simulink model "SMC_for_takeoff"  (R2018b)
settings: Solver=ode45  StartTime=0.0  StopTime=10.0  RelTol=1e-3
libraries: simulink x3
settings Model: Creator=mchehadeh  LastModifiedBy=aaa_b
settings DataIOCC: LimitDataPoints=on  SaveFormat=Array  SignalLoggingSaveFormat=ModelDataLogs
settings OptimizationCC: BlockReduction=off  BooleanDataType=off  ExpressionDepthLimit=2147483647  LifeSpan=inf
settings DebuggingCC: SaveWithParameterizedLinksMsg=none  UnderspecifiedInitializationDetection=Classic  MergeDetectMultiDrivingBlocksExec=none  SignalResolutionControl=TryResolveAllWithWarning  MultiTaskDSMMsg=warning  MultiTaskCondExecSysMsg=none  StateNameClashWarn=warning  SFUnexpectedBacktrackingDiag=warning  SFNoUnconditionalDefaultTransitionDiag=warning  SFExecutionAtInitializationDiag=none
settings HardwareCC: ProdBitPerPointer=32  ProdBitPerSizeT=32  ProdBitPerPtrDiffT=32  ProdLargestAtomicFloat=None  ProdIntDivRoundTo=Undefined  ProdEndianess=Unspecified  ProdWordSize=32  ProdHWDeviceType=32-bit Generic  TargetUnknown=on
settings ModelReferenceCC: PropagateSignalLabelsOutOfModel=off
settings SFSimCC: SimUseLocalCustomCode=off
settings RTWCC: RTWUseLocalCustomCode=off
settings CodeAppCC: StateflowObjectComments=on
settings GRTTargetCC: TargetLangStandard=C89/C90 (ANSI)  GeneratePreprocessorConditionals=Disable all
settings ConfigComp: CovMetricSettings=dw  CovHtmlReporting=on  CovSaveCumulativeToWorkspaceVar=on  CovSaveSingleToWorkspaceVar=on  CovExternalEMLEnable=off

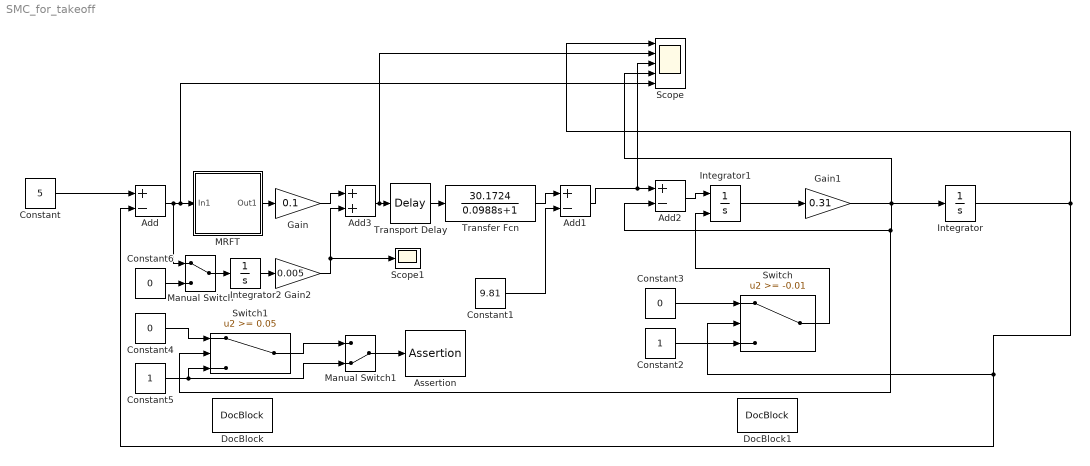
== system SMC_for_takeoff ==
  Add : Sum  Inputs=+-
  Add1 : Sum  Inputs=+-
  Add2 : Sum  Inputs=+-
  Add3 : Sum
  Assertion : Assertion  AssertionFailFcn=|  StopWhenAssertionFail=off
      | set_param(bdroot,'SimulationCommand','pause'),
      | disp(sprintf('\nSimulation paused.'))
  Constant : Constant  Value=5
  Constant1 : Constant  Value=9.81
  Constant2 : Constant
  Constant3 : Constant  Value=0
  Constant4 : Constant  Value=0
  Constant5 : Constant
  Constant6 : Constant  Value=0
  DocBlock : simulink/Model-Wide Utilities/DocBlock  DocumentType=Text
  DocBlock1 : simulink/Model-Wide Utilities/DocBlock  DocumentType=Text
  Gain : Gain  Gain=0.1
  Gain1 : Gain  Gain=0.31
  Gain2 : Gain  Gain=0.005
  Integrator : Integrator  LimitOutput=on  LowerSaturationLimit=0
  Integrator1 : Integrator  ExternalReset=level  LowerSaturationLimit=0
  Integrator2 : Integrator
  MRFT : Subsystem
  Manual Switch : ManualSwitch
  Manual Switch1 : ManualSwitch  CurrentSetting=0
  Scope : Scope  NumInputPorts=5
  Scope1 : Scope
  Switch : Switch  Threshold=-0.01
  Switch1 : Switch  Threshold=0.05
  Transfer Fcn : TransferFcn  Numerator=[30.1724]  Denominator=[0.0988 1]
  Transport Delay : TransportDelay  DelayTime=0.0709
  wires:
  Transport Delay/1 -> Transfer Fcn/1
  Integrator/1 -> Switch/2, Add/2, Scope/1
  MRFT/1(Out1) -> Gain/1
  Transfer Fcn/1 -> Add1/1
  Constant/1 -> Add/1
  Constant1/1 -> Add1/2
  Add1/1 -> Add2/1, Scope/3
  Constant2/1 -> Switch/3
  Integrator1/1 -> Gain1/1
  Gain1/1 -> Switch1/2, Add2/2, Scope/4, Integrator/1
  Constant3/1 -> Switch/1
  Add2/1 -> Integrator1/1
  Switch/1 -> Integrator1/2
  Add/1 -> Manual Switch/1, Scope/5, MRFT/1(In1)
  Integrator2/1 -> Gain2/1
  Add3/1 -> Scope/2, Transport Delay/1
  Gain/1 -> Add3/1
  Gain2/1 -> Add3/2, Scope1/1
  Constant4/1 -> Switch1/1
  Constant5/1 -> Manual Switch1/2, Switch1/3
  Manual Switch/1 -> Integrator2/1
  Constant6/1 -> Manual Switch/2
  Manual Switch1/1 -> Assertion/1
  Switch1/1 -> Manual Switch1/1

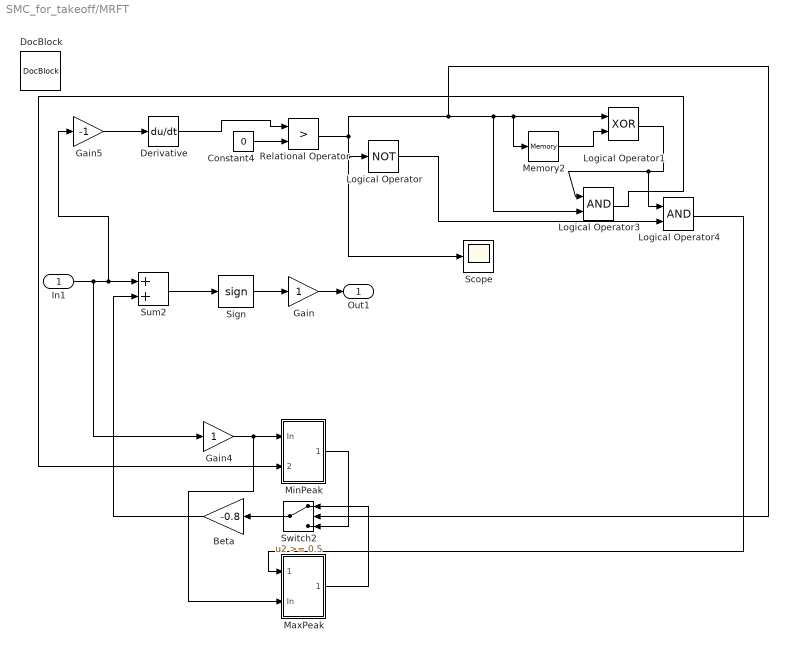
== system SMC_for_takeoff/MRFT ==
  In1 : Inport
  Beta : Gain  Gain=-0.8  SaturateOnIntegerOverflow=on  OutDataTypeStr=Inherit: Same as input  ParamDataTypeStr=Inherit: Same as input
  Constant4 : Constant  Value=0
  Derivative : Derivative  CoefficientInTFapproximation=0.0002
  DocBlock : simulink/Model-Wide Utilities/DocBlock  DocumentType=Text
  Gain : Gain  SaturateOnIntegerOverflow=on  OutDataTypeStr=Inherit: Same as input  ParamDataTypeStr=Inherit: Same as input
  Gain4 : Gain  SaturateOnIntegerOverflow=on  OutDataTypeStr=Inherit: Same as input  ParamDataTypeStr=Inherit: Same as input
  Gain5 : Gain  Gain=-1  SaturateOnIntegerOverflow=on  OutDataTypeStr=Inherit: Same as input  ParamDataTypeStr=Inherit: Same as input
  Logical Operator : Logic  Operator=NOT  Inputs=1
  Logical Operator1 : Logic  Operator=XOR
  Logical Operator3 : Logic
  Logical Operator4 : Logic
  MaxPeak : Subsystem
  Memory2 : Memory
  MinPeak : Subsystem
  Relational Operator : RelationalOperator  Operator=>  RndMeth=Nearest  InputSameDT=on
  Scope : Scope
  Sign : Signum
  Sum2 : Sum  SaturateOnIntegerOverflow=on  InputSameDT=on  OutDataTypeStr=Inherit: Same as first input
  Switch2 : Switch  Threshold=0.5  SaturateOnIntegerOverflow=on  InputSameDT=on
  Out1 : Outport
  wires:
  Memory2/1 -> Logical Operator1/2
  Switch2/1 -> Beta/1
  Logical Operator1/1 -> Logical Operator4/1, Logical Operator3/1
  Logical Operator4/1 -> MaxPeak/1(Cntrl)
  Constant4/1 -> Relational Operator/2
  Relational Operator/1 -> Scope/1, Logical Operator/1, Logical Operator1/1, Memory2/1, Logical Operator3/2, Switch2/2
  Logical Operator3/1 -> MinPeak/2(Cntrl)
  Logical Operator/1 -> Logical Operator4/2
  Sign/1 -> Gain/1
  Gain4/1 -> MinPeak/1(In), MaxPeak/2(In)
  Sum2/1 -> Sign/1
  In1/1 -> Gain4/1, Gain5/1, Sum2/1
  Beta/1 -> Sum2/2
  MaxPeak/1(Out) -> Switch2/1
  MinPeak/1(Out) -> Switch2/3
  Gain5/1 -> Derivative/1
  Derivative/1 -> Relational Operator/1
  Gain/1 -> Out1/1

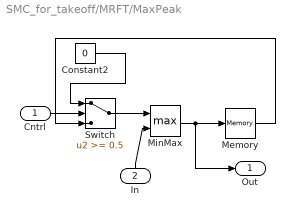
== system SMC_for_takeoff/MRFT/MaxPeak ==
  Cntrl : Inport
  In : Inport  Port=2
  Constant2 : Constant  Value=0
  Memory : Memory
  MinMax : MinMax  Function=max  Inputs=2  SaturateOnIntegerOverflow=on  InputSameDT=on
  Switch : Switch  Threshold=0.5  SaturateOnIntegerOverflow=on  InputSameDT=on
  Out : Outport
  wires:
  MinMax/1 -> Memory/1, Out/1
  Switch/1 -> MinMax/1
  Constant2/1 -> Switch/1
  Memory/1 -> Switch/3
  In/1 -> MinMax/2
  Cntrl/1 -> Switch/2

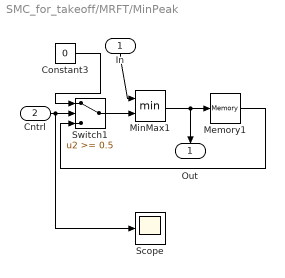
== system SMC_for_takeoff/MRFT/MinPeak ==
  In : Inport
  Cntrl : Inport  Port=2
  Constant3 : Constant  Value=0
  Memory1 : Memory
  MinMax1 : MinMax  Inputs=2  SaturateOnIntegerOverflow=on  InputSameDT=on
  Scope : Scope
  Switch1 : Switch  Threshold=0.5  SaturateOnIntegerOverflow=on  InputSameDT=on
  Out : Outport
  wires:
  MinMax1/1 -> Memory1/1, Out/1
  Switch1/1 -> MinMax1/2
  Memory1/1 -> Switch1/3
  Constant3/1 -> Switch1/1
  In/1 -> MinMax1/1
  Cntrl/1 -> Switch1/2, Scope/1
